simulink model "SimTrackFollowing"  (Simulink 5.1)
settings: Solver=ode45  StartTime=0.0  StopTime=NmaxTs*Ts  FixedStep=Tc/10  RelTol=1e-3
values from neighbouring files (symbols this model uses):
  g_flutter = 1    [followdemo.m]
  g_rro = 1    [followdemo.m]
  g_sensor = 1    [followdemo.m]
  g_torque = 1    [followdemo.m]
  loopgain = 1+loopgain_pt(jj)    [evperf.m]
  Tc = Ts/2    [followdemo.m]
  Ts = PlantData.Ts    [followdemo.m]
undefined symbols (not defined in the file or in its folder): FlutterDist, ForceDist, RRO, SensorNoise
libraries: cstblocks x3
settings Model: LastModifiedBy=takeyori  BooleanDataType=on  ProdHWDeviceType=Microprocessor

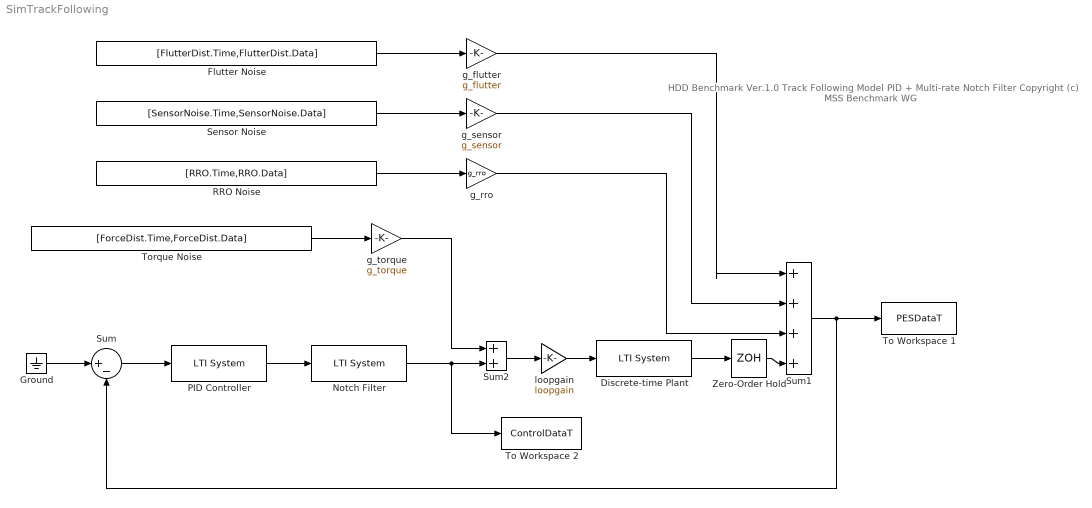
== system SimTrackFollowing ==
  note: HDD Benchmark Ver.1.0
      | Track Following Model
      | PID + Multi-rate Notch Filter
      | Copyright (c) MSS Benchmark WG
  Discrete-time Plant : cstblocks/LTI System  sys=sysd_P  IC=0
  Flutter Noise : FromWorkspace  VariableName=[FlutterDist.Time,FlutterDist.Data]  SampleTime=FlutterDist.Ts  Interpolate=off  OutputAfterFinalValue=Setting to zero
  Ground : Ground
  Notch Filter : cstblocks/LTI System  sys=sys_C2  IC=0
  PID Controller : cstblocks/LTI System  sys=sys_C1  IC=[]
  RRO Noise : FromWorkspace  VariableName=[RRO.Time,RRO.Data]  SampleTime=RRO.Ts  Interpolate=off  OutputAfterFinalValue=Setting to zero
  Sensor Noise : FromWorkspace  VariableName=[SensorNoise.Time,SensorNoise.Data]  SampleTime=SensorNoise.Ts  Interpolate=off  OutputAfterFinalValue=Setting to zero
  Sum : Sum  Inputs=|+-  ShowAdditionalParam=on  SaturateOnIntegerOverflow=on
  Sum1 : Sum  Inputs=+++|+  SaturateOnIntegerOverflow=on
  Sum2 : Sum  ShowAdditionalParam=on  SaturateOnIntegerOverflow=on
  To Workspace 1 : ToWorkspace  VariableName=PESDataT  SampleTime=Ts  SaveFormat=StructureWithTime
      settings: MaxDataPoints=NmaxTs
  To Workspace 2 : ToWorkspace  VariableName=ControlDataT  SampleTime=Tc  SaveFormat=StructureWithTime
      settings: MaxDataPoints=NmaxTc
  Torque Noise : FromWorkspace  VariableName=[ForceDist.Time,ForceDist.Data]  SampleTime=ForceDist.Ts  Interpolate=off  OutputAfterFinalValue=Setting to zero
  Zero-Order Hold : ZeroOrderHold  SampleTime=Ts
  g_flutter : Gain  Gain=g_flutter  SaturateOnIntegerOverflow=on
  g_rro : Gain  Gain=g_rro  SaturateOnIntegerOverflow=on
  g_sensor : Gain  Gain=g_sensor  SaturateOnIntegerOverflow=on
  g_torque : Gain  Gain=g_torque  SaturateOnIntegerOverflow=on
  loopgain : Gain  Gain=loopgain  SaturateOnIntegerOverflow=on
  wires:
  Ground/1 -> Sum/1
  Sum/1 -> PID Controller/1
  Notch Filter/1 -> Sum2/2, To Workspace 2/1
  Sum1/1 -> Sum/2, To Workspace 1/1
  g_torque/1 -> Sum2/1
  Torque Noise/1 -> g_torque/1
  Sensor Noise/1 -> g_sensor/1
  g_sensor/1 -> Sum1/2
  Flutter Noise/1 -> g_flutter/1
  g_flutter/1 -> Sum1/1
  RRO Noise/1 -> g_rro/1
  g_rro/1 -> Sum1/3
  Sum2/1 -> loopgain/1
  loopgain/1 -> Discrete-time Plant/1
  Discrete-time Plant/1 -> Zero-Order Hold/1
  Zero-Order Hold/1 -> Sum1/4
  PID Controller/1 -> Notch Filter/1
